simulink model "pole_assigment"  (R2020b)
settings: Solver=VariableStepAuto  StartTime=0.0  StopTime=10.0  RelTol=1e-3
settings Model: Creator=petir  LastModifiedBy=petir

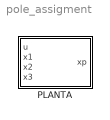
== system pole_assigment ==
  PLANTA : MATLAB Function  TreatAsAtomicUnit=on

== matlab function pole_assigment/PLANTA ==
  data: u input; xp output; x1 input; x2 input; x3 input
function xp = fcn(u, x1, x2, x3)
% Parametros
A = [0 1 0; 0 0 1; -1 -5 -6]
B = [0; 0; 1];
% Vector 
x = [x1; x2; x3;]

% Planta
xp = A * x + B * u;
